simulink model "Control_try_final_2020b"  (R2020b)
settings: Solver=VariableStepAuto  StartTime=0.0  StopTime=inf  RelTol=1e-3
undefined symbols (not defined in the file or in its folder): DiscIntNeverNeededParam
libraries: mobileRoboticsLib x25
(part 3 of 7)

== system Control_try_final_2020b/Team_1_behaviour/T1R3 (defender 1)/Team 1 Behaviour ==
  Ball Loc : Inport
  Robot 1 T1 Loc : Inport  Port=2
  Angle Finder : Subsystem
  Chart : Stateflow chart  TreatAsAtomicUnit=on
      settings: PortSchema="{\"entries\":[{\"content\":{\"sides\":[{\"content\":{\"connectorIds\":[\"In5\",\"In1\",\"In2\",\"In3\",\"In4\",\"In6\"]},\"type\":\"ConnectorPlacement.EquallySpacedRectSide\",\"uuid\":\"cd25ea97-6441-4246-83f2-eec847899c89\"},{\"content\":{\"connectorIds\":[\"Out1\"],\"side\":\"RIGHT\"},\"type\":\"ConnectorPlacement.EquallySpacedRectSide\",\"uuid\":\"ef7d77a7-1549-4474-8b84-35bb8af5d0e7\"},{\"content\":{\"connectorIds\":[],\"side\":\"TOP\"},\"type\":\"ConnectorPlacement.EquallySpacedRectSide\",\"uuid\":\"0f0ce596-3061-42ac-890a-62bc4f21ac3e\"},{\"content\":{\"connectorIds\":[],\"side\":\"BOTTOM\"},\"type\":\"ConnectorPlacement.EquallySpacedRectSide\",\"uuid\":\"682b3de5-e999-4954-b7ff-f16ecbf9ea8f\"}]},\"type\":\"ConnectorPlacement.EquallySpacedConnector\",\"uuid\":\"15dca8e2-6a60-4a0d-80a5-3c295a61c828\"}],\"packageUris\":[\"http://schema.mathworks.com/mf0/Connector/R2020b\"],\"version\":\"1.0\"}"
  Chart3 : Stateflow chart  TreatAsAtomicUnit=on
  Constant : Constant  Value=10
  Constant1 : Constant  Value=4
  Constant2 : Constant  Value=2
  Constant3 : Constant  Value=0
  Demux1 : Demux  Outputs=3
  Demux3 : Demux  Outputs=3
  Matrix Concatenate : Concatenate  Mode=Multidimensional array  ConcatenateDimension=2
  Mod : Math  Operator=mod  SaturateOnIntegerOverflow=on
  Pi : Constant  Value=pi  OutDataTypeStr=Inherit: Inherit via back propagation
  Product1 : Product
  Proximity_Finder_Ball : Subsystem
  Sum : Sum  Inputs=+-
  Sum1 : Sum  Inputs=-+
  Vector Concatenate : Concatenate
  Vector Concatenate1 : Concatenate  NumInputs=3
  Vector Concatenate2 : Concatenate
  Velocity_Decider : Stateflow chart  TreatAsAtomicUnit=on
  kick_direction : Subsystem
  XYZK : Outport
  VxVyW : Outport  Port=2
  wires:
  Ball Loc/1 -> Demux3/1
  Sum/1 -> Proximity_Finder_Ball/1(In1), Angle Finder/1(In1)
  Robot 1 T1 Loc/1 -> Demux1/1
  Demux1/1 -> Matrix Concatenate/1, Chart/3(Rx)
  Demux1/2 -> Matrix Concatenate/2, Chart/4(Ry)
  Matrix Concatenate/1 -> Sum1/2, Sum/1
  Demux3/2 -> Vector Concatenate2/2, Chart/2(By)
  Demux3/1 -> Vector Concatenate2/1, Chart/1(Bx)
  Demux1/3 -> Mod/1
  Pi/1 -> Product1/1
  Constant2/1 -> Product1/2
  Product1/1 -> Mod/2
  Chart/1(actual_angle) -> Chart3/2(DT)
  Mod/1 -> Chart/6(angle_bot)
  Angle Finder/1(angle) -> Chart/5(angle)
  Proximity_Finder_Ball/1(DBR) -> Velocity_Decider/1(DBR)
  Velocity_Decider/2(velocity) -> Chart3/1(velocity)
  Constant/1 -> Vector Concatenate/1
  Constant1/1 -> Vector Concatenate/2
  Vector Concatenate/1 -> Sum1/1
  Sum1/1 -> kick_direction/1(In1)
  Velocity_Decider/1(kick) -> kick_direction/2(kick)
  kick_direction/1(Out1) -> XYZK/1
  Chart3/1(v) -> Vector Concatenate1/1
  Chart3/2(w) -> Vector Concatenate1/3
  Constant3/1 -> Vector Concatenate1/2
  Vector Concatenate1/1 -> VxVyW/1
  Vector Concatenate2/1 -> Sum/2

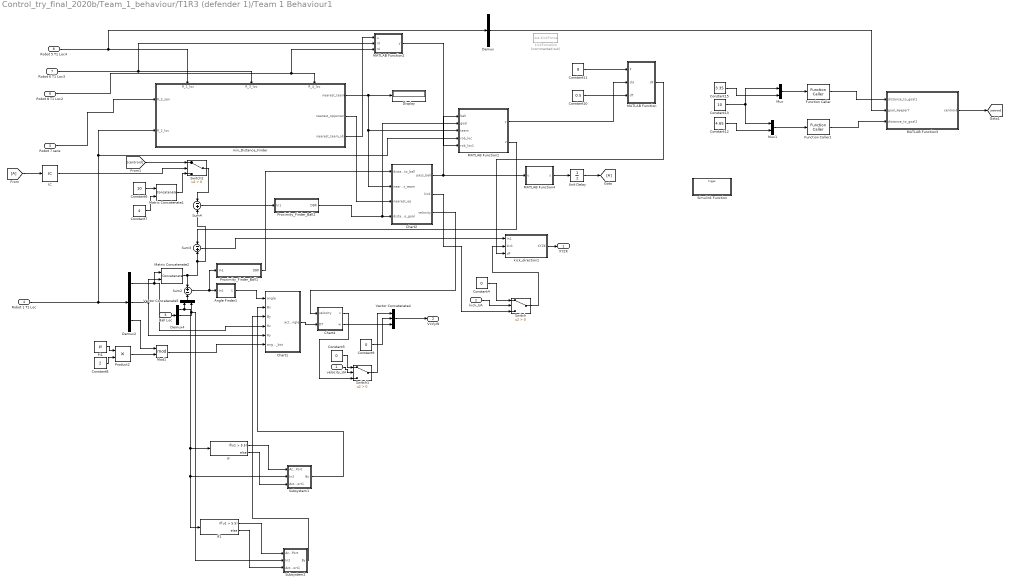
== system Control_try_final_2020b/Team_1_behaviour/T1R3 (defender 1)/Team 1 Behaviour1 ==
  velocity_UA : Inport
  kick_UA : Inport  Port=2
  Ball Loc : Inport  Port=3
  Robot 1 T1 Loc : Inport  Port=4
  Robot 7 sens : Inport  Port=5
  Robot 8 T1 Loc2 : Inport  Port=6
  Robot 6 T1 Loc3 : Inport  Port=7
  Robot 5 T1 Loc4 : Inport  Port=8
  Angle Finder1 : Subsystem
  Chart1 : Stateflow chart  TreatAsAtomicUnit=on
      settings: PortSchema="{\"entries\":[{\"content\":{\"sides\":[{\"content\":{\"connectorIds\":[\"In5\",\"In1\",\"In2\",\"In3\",\"In4\",\"In6\"]},\"type\":\"ConnectorPlacement.EquallySpacedRectSide\",\"uuid\":\"cd25ea97-6441-4246-83f2-eec847899c89\"},{\"content\":{\"connectorIds\":[\"Out1\"],\"side\":\"RIGHT\"},\"type\":\"ConnectorPlacement.EquallySpacedRectSide\",\"uuid\":\"ef7d77a7-1549-4474-8b84-35bb8af5d0e7\"},{\"content\":{\"connectorIds\":[],\"side\":\"TOP\"},\"type\":\"ConnectorPlacement.EquallySpacedRectSide\",\"uuid\":\"0f0ce596-3061-42ac-890a-62bc4f21ac3e\"},{\"content\":{\"connectorIds\":[],\"side\":\"BOTTOM\"},\"type\":\"ConnectorPlacement.EquallySpacedRectSide\",\"uuid\":\"682b3de5-e999-4954-b7ff-f16ecbf9ea8f\"}]},\"type\":\"ConnectorPlacement.EquallySpacedConnector\",\"uuid\":\"15dca8e2-6a60-4a0d-80a5-3c295a61c828\"}],\"packageUris\":[\"http://schema.mathworks.com/mf0/Connector/R2020b\"],\"version\":\"1.0\"}"
  Chart2 : Stateflow chart  TreatAsAtomicUnit=on
      settings: PortSchema="{\"entries\":[{\"content\":{\"sides\":[{\"content\":{\"connectorIds\":[\"In1\",\"In2\",\"In3\",\"In4\"]},\"type\":\"ConnectorPlacement.EquallySpacedRectSide\",\"uuid\":\"0588d813-8053-43c2-aa9d-d3a846613814\"},{\"content\":{\"connectorIds\":[\"Out3\",\"Out1\",\"Out2\"],\"side\":\"RIGHT\"},\"type\":\"ConnectorPlacement.EquallySpacedRectSide\",\"uuid\":\"b273383a-6a54-4b9f-9eb1-40fc7adfc00e\"},{\"content\":{\"connectorIds\":[],\"side\":\"TOP\"},\"type\":\"ConnectorPlacement.EquallySpacedRectSide\",\"uuid\":\"d9b37716-6c8a-415a-a248-7c4c2a5acdca\"}]},\"type\":\"ConnectorPlacement.EquallySpacedConnector\",\"uuid\":\"4383e6fa-6fc5-4afb-a6cc-0c4f83dd9bd6\"}],\"packageUris\":[\"http://schema.mathworks.com/mf0/Connector/R2020b\"],\"version\":\"1.0\"}"
  Chart4 : Stateflow chart  TreatAsAtomicUnit=on
  Constant10 : Constant  Value=0.5
  Constant11 : Constant  Value=8
  Constant12 : Constant  Value=4.65
  Constant13 : Constant  Value=10
  Constant15 : Constant  Value=3.35
  Constant4 : Constant  Value=0
  Constant5 : Constant  Value=0
  Constant6 : Constant  Value=10
  Constant7 : Constant  Value=4
  Constant8 : Constant  Value=2
  Constant9 : Constant  Value=0
  Demux : Demux  Outputs=3
  Demux2 : Demux  Outputs=3
  Demux4 : Demux  Outputs=3
  Display : Display
  Function Caller : FunctionCaller  FunctionPrototype=y = f(u)  InputArgumentSpecifications=<Enter example>  OutputArgumentSpecifications=<Enter example>
  Function Caller1 : FunctionCaller  FunctionPrototype=y = f(u)  InputArgumentSpecifications=<Enter example>  OutputArgumentSpecifications=<Enter example>
  IC : InitialCondition  Value=0
  If : If  IfExpression=u1 > 5.5
  If1 : If  IfExpression=u1 > 5.5
  MATLAB Function : MATLAB Function  TreatAsAtomicUnit=on
  MATLAB Function1 : MATLAB Function  TreatAsAtomicUnit=on
  MATLAB Function2 : MATLAB Function  TreatAsAtomicUnit=on
  MATLAB Function3 : MATLAB Function  TreatAsAtomicUnit=on
  MATLAB Function4 : MATLAB Function  TreatAsAtomicUnit=on
  Matrix Concatenate1 : Concatenate  Mode=Multidimensional array  ConcatenateDimension=2
  Matrix Concatenate2 : Concatenate  Mode=Multidimensional array  ConcatenateDimension=2
  Mod1 : Math  Operator=mod  SaturateOnIntegerOverflow=on
  Mux : Mux  Inputs=2
  Mux1 : Mux  Inputs=2
  Pi1 : Constant  Value=pi  OutDataTypeStr=Inherit: Inherit via back propagation
  Product2 : Product
  Proximity_Finder_Ball1 : Subsystem
  Proximity_Finder_Ball2 : Subsystem
  Simulink Function : Subsystem  TreatAsAtomicUnit=on
  Subsystem1 : Subsystem
  Subsystem2 : Subsystem
  Sum2 : Sum  Inputs=+-
  Sum3 : Sum  Inputs=-+
  Sum4 : Sum  Inputs=-+
  Switch : Switch  Criteria=u2 > Threshold
  Switch1 : Switch  Criteria=u2 > Threshold
  Switch2 : Switch  Criteria=u2 > Threshold
  Unit Delay : UnitDelay  SampleTime=-1  HasFrameUpgradeWarning=on
  Vector Concatenate4 : Concatenate  NumInputs=3
  Vector Concatenate5 : Concatenate
  kickForceSim : FromWorkspace  Commented=on  VariableName=out.KickForce
  kick_direction1 : Subsystem
  min_Distance_Finder : Subsystem
      settings: PortSchema="{\"entries\":[{\"content\":{\"sides\":[{\"content\":{\"connectorIds\":[\"In1\",\"In2\"]},\"type\":\"ConnectorPlacement.EquallySpacedRectSide\",\"uuid\":\"45cf91c7-7d38-4a19-bf35-d1d31095287a\"},{\"content\":{\"connectorIds\":[\"Out1\",\"Out2\",\"Out3\"],\"side\":\"RIGHT\"},\"type\":\"ConnectorPlacement.EquallySpacedRectSide\",\"uuid\":\"645394ba-2e5d-4060-b61c-cc9330ee0038\"},{\"content\":{\"connectorIds\":[\"In3\",\"In4\",\"In5\"],\"side\":\"TOP\"},\"type\":\"ConnectorPlacement.EquallySpacedRectSide\",\"uuid\":\"4fc56b73-04ec-476f-b487-f0e593f708ad\"},{\"content\":{\"connectorIds\":[],\"side\":\"BOTTOM\"},\"type\":\"ConnectorPlacement.EquallySpacedRectSide\",\"uuid\":\"cd306436-fd63-4e79-88e6-7a63c0840ed7\"}]},\"type\":\"ConnectorPlacement.EquallySpacedConnector\",\"uuid\":\"5cf2ee04-00eb-490b-958c-5fb90b43d325\"}],\"packageUris\":[\"http://schema.mathworks.com/mf0/Connector/R2020b\"],\"version\":\"1.0\"}"
  XYZK : Outport
  VxVyW : Outport  Port=2
  wires:
  Constant4/1 -> Switch/1
  kick_UA/1 -> Switch/2
  Constant5/1 -> Switch1/1
  velocity_UA/1 -> Switch1/2
  MATLAB Function4/1(y) -> Unit Delay/1
  If1/2 -> Subsystem2/3(Action Port1)
  Constant6/1 -> Matrix Concatenate1/1
  Constant9/1 -> Vector Concatenate4/2
  Demux4/1 -> If1/1, Subsystem1/2(In2), If/1, Vector Concatenate5/1
  Matrix Concatenate2/1 -> Sum4/2, Sum3/2, Sum2/1
  Chart1/1(actual_angle) -> Chart4/2(DT)
  Subsystem1/1(Bx) -> Chart1/1(Bx)
  Demux2/3 -> Mod1/1
  Constant8/1 -> Product2/2
  If/2 -> Subsystem1/3(Action Port1)
  Sum3/1 -> kick_direction1/1(In1)
  Robot 6 T1 Loc3/1 -> MATLAB Function2/2(r3), min_Distance_Finder/4(R_3_loc)
  Demux4/2 -> Subsystem2/2(In2), Vector Concatenate5/2
  Proximity_Finder_Ball2/1(DBR) -> MATLAB Function1/2(goal), Chart2/4(distance_to_goal)
  min_Distance_Finder/3(nearest_team_idx) -> MATLAB Function2/1(u)
  If1/1 -> Subsystem2/1(Action Port)
  If/1 -> Subsystem1/1(Action Port)
  Pi1/1 -> Product2/1
  Function Caller1/1 -> MATLAB Function3/3(distance_to_goal2)
  Chart4/2(w) -> Vector Concatenate4/3
  Ball Loc/1 -> Demux4/1
  Robot 8 T1 Loc2/1 -> MATLAB Function2/3(r4), min_Distance_Finder/5(R_4_loc)
  [A] -> IC/1
  kick_direction1/1(XYZK) -> XYZK/1
  Robot 7 sens/1 -> min_Distance_Finder/1(R_2_sen)
  Constant15/1 -> Mux/2
  Mod1/1 -> Chart1/6(angle_bot)
  Sum2/1 -> Proximity_Finder_Ball1/1(In1), Angle Finder1/1(In1)
  Robot 1 T1 Loc/1 -> MATLAB Function1/4(rob_loc), min_Distance_Finder/2(R_2_loc), Demux2/1
  Demux/2 -> MATLAB Function3/2(goal_keeperY)
  Constant13/1 -> Mux1/1, Mux/1
  MATLAB Function1/1(y) -> MATLAB Function/2(dis)
  Demux2/2 -> Matrix Concatenate2/2, Chart1/4(Ry)
  MATLAB Function1/2(z) -> Sum3/1
  Unit Delay/1 -> [A]
  Chart2/3(pass_beh) -> MATLAB Function1/1(beh), MATLAB Function4/1(u)
  Vector Concatenate4/1 -> VxVyW/1
  Constant12/1 -> Mux1/2
  Proximity_Finder_Ball1/1(DBR) -> Chart2/1(distance_to_ball)
  Mux1/1 -> Function Caller1/1
  Mux/1 -> Function Caller/1
  Constant10/1 -> MATLAB Function/3(dT)
  Sum4/1 -> Proximity_Finder_Ball2/1(In1)
  MATLAB Function3/1(centroid) -> [centroid]
  Switch2/1 -> Sum4/1
  min_Distance_Finder/1(nearest_team) -> Chart2/2(nearest_team), MATLAB Function1/3(team), Display/1
  min_Distance_Finder/2(nearest_opponent) -> Chart2/3(nearest_op)
  Chart4/1(v) -> Switch1/3
  Chart2/2(velocity) -> Chart4/1(velocity)
  Subsystem2/1(By) -> Chart1/2(By)
  Chart2/1(kick) -> Switch/3
  Function Caller/1 -> MATLAB Function3/1(distance_to_goal1)
  Angle Finder1/1(angle) -> Chart1/5(angle)
  Product2/1 -> Mod1/2
  MATLAB Function/1(dF) -> kick_direction1/3(dF)
  Matrix Concatenate1/1 -> Switch2/3
  Robot 5 T1 Loc4/1 -> Demux/1, min_Distance_Finder/3(R_1_loc)
  MATLAB Function2/1(y) -> MATLAB Function1/5(rob_loc1)
  Constant11/1 -> MATLAB Function/1(F)
  Demux2/1 -> Matrix Concatenate2/1, Chart1/3(Rx)
  Constant7/1 -> Matrix Concatenate1/2
  IC/1 -> Switch2/2
  Vector Concatenate5/1 -> Sum2/2
  [centroid] -> Switch2/1
  Switch/1 -> kick_direction1/2(kick)
  Switch1/1 -> Vector Concatenate4/1

== system Control_try_final_2020b/Team_2_Behaviour/T2_R1(Goal_Keeper)/Distance ==
  In1 : Inport
  In2 : Inport  Port=2
  In3 : Inport  Port=3
  In4 : Inport  Port=4
  Square : Math  Operator=square  SaturateOnIntegerOverflow=on
  Square Root : Sqrt  SaturateOnIntegerOverflow=on
  Square1 : Math  Operator=square  SaturateOnIntegerOverflow=on
  Sum : Sum  Inputs=|+-
  Sum1 : Sum  Inputs=|+-
  Sum2 : Sum  Inputs=|++
  GB_dist : Outport
  wires:
  Square1/1 -> Sum2/2
  Sum2/1 -> Square Root/1
  Square/1 -> Sum2/1
  Sum1/1 -> Square1/1
  Sum/1 -> Square/1
  In1/1 -> Sum/1
  In3/1 -> Sum/2
  In2/1 -> Sum1/1
  In4/1 -> Sum1/2
  Square Root/1 -> GB_dist/1

== system Control_try_final_2020b/Team_2_Behaviour/T2_R1(Goal_Keeper)/angle_finder ==
  kick_direction : Inport
  R_1_loc : Inport  Port=2
  kick : Inport  Port=3
  Atan : Trigonometry  Operator=atan
  Constant : Constant  Value=2.5
  Constant1 : Constant  Value=-2.5
  Constant2 : Constant  Value=0
  Constant3 : Constant  Value=-1
  Cos : Trigonometry  Operator=cos
  Demux : Demux  Outputs=3
  Divide : Product  Inputs=/*
  Product : Product  Inputs=3
  Product1 : Product
  Sin : Trigonometry
  Sum : Sum  Inputs=|+-
  Vector Concatenate : Concatenate  NumInputs=4
  Out1 : Outport
  wires:
  kick_direction/1 -> Sum/1
  R_1_loc/1 -> Sum/2
  Sum/1 -> Demux/1
  Demux/1 -> Divide/1
  Demux/2 -> Divide/2
  Divide/1 -> Atan/1
  Atan/1 -> Cos/1, Sin/1
  Constant/1 -> Product/2
  Cos/1 -> Product/3
  Sin/1 -> Product1/1
  Constant1/1 -> Product1/2
  Vector Concatenate/1 -> Out1/1
  kick/1 -> Vector Concatenate/4
  Constant2/1 -> Vector Concatenate/3
  Product1/1 -> Vector Concatenate/2
  Product/1 -> Vector Concatenate/1
  Constant3/1 -> Product/1

== system Control_try_final_2020b/Team_2_Behaviour/T2_R1(Goal_Keeper)/min_Distance_Finder ==
  R_1_sen : Inport
  R_1_loc : Inport  Port=2
  R_2_loc : Inport  Port=3
  R_3_loc : Inport  Port=4
  R_4_loc : Inport  Port=5
  Display{,1..2,4} (4 alike) : Display
  Distance : Subsystem
  Distance1 : Subsystem
  Distance2 : Subsystem
  Kick_prob_calc : Stateflow chart  TreatAsAtomicUnit=on
      settings: PortSchema="{\"entries\":[{\"content\":{\"sides\":[{\"content\":{\"connectorIds\":[\"In4\",\"In5\",\"In6\"]},\"type\":\"ConnectorPlacement.EquallySpacedRectSide\",\"uuid\":\"64545375-395a-4478-8a53-b77c7ccd5016\"},{\"content\":{\"connectorIds\":[\"Out1\"],\"side\":\"RIGHT\"},\"type\":\"ConnectorPlacement.EquallySpacedRectSide\",\"uuid\":\"7cc0c28a-cc26-4f23-9952-6261e736221a\"},{\"content\":{\"connectorIds\":[\"In2\",\"In3\",\"In1\"],\"side\":\"TOP\"},\"type\":\"ConnectorPlacement.EquallySpacedRectSide\",\"uuid\":\"3f39c863-1804-4707-87c1-6f77798d874b\"},{\"content\":{\"connectorIds\":[],\"side\":\"BOTTOM\"},\"type\":\"ConnectorPlacement.EquallySpacedRectSide\",\"uuid\":\"dd00a5df-2ac1-49a5-bc9d-cbc3bc53305b\"}]},\"type\":\"ConnectorPlacement.EquallySpacedConnector\",\"uuid\":\"731ad359-9b43-4c19-839e-d6f1a372c8a6\"}],\"packageUris\":[\"http://schema.mathworks.com/mf0/Connector/R2020b\"],\"version\":\"1.0\"}"
  Multiply : Gain  Gain=2
  Multiply1 : Gain  Gain=2
  Multiply2 : Gain  Gain=2
  R2_O_dist_val : Subsystem
  R3_O_dist_val : Subsystem
  R4_O_dist_val : Subsystem
  Sum : Sum  Inputs=|--
  Sum1 : Sum  Inputs=|--
  Sum2 : Sum  Inputs=|--
  zero_padding : MATLAB Function  TreatAsAtomicUnit=on
  kick_direction : Outport
  wires:
  R_2_loc/1 -> R2_O_dist_val/2(R_2_loc), Distance/2(R_2_loc), Kick_prob_calc/2(R_2_loc)
  R_1_loc/1 -> R4_O_dist_val/1(R_1_loc), R3_O_dist_val/1(R_1_loc), R2_O_dist_val/1(R_1_loc), Distance2/1(R_1_loc), Distance1/1(R_1_loc), Distance/1(R_1_loc)
  R_3_loc/1 -> R3_O_dist_val/2(R_2_loc), Distance1/2(R_3_loc), Kick_prob_calc/3(R_3_loc)
  R_4_loc/1 -> R4_O_dist_val/2(R_2_loc), Distance2/2(R_4_loc), Kick_prob_calc/1(R_4_loc)
  Kick_prob_calc/1(kick_direction) -> Display4/1, kick_direction/1
  R_1_sen/1 -> zero_padding/1(u)
  zero_padding/1(y) -> R3_O_dist_val/3(sen_1_val), R4_O_dist_val/3(sen_1_val), R2_O_dist_val/3(sen_1_val)
  R2_O_dist_val/1(y) -> Display/1, Multiply1/1
  R3_O_dist_val/1(y) -> Display1/1, Multiply2/1
  R4_O_dist_val/1(y) -> Display2/1, Multiply/1
  Distance/1(R1_R2_dis) -> Sum/1
  Multiply1/1 -> Sum/2
  Distance1/1(R1_R3_dis) -> Sum1/1
  Distance2/1(R1_R4_dis) -> Sum2/1
  Multiply2/1 -> Sum1/2
  Multiply/1 -> Sum2/2
  Sum/1 -> Kick_prob_calc/4(R1_R2_dis)
  Sum1/1 -> Kick_prob_calc/5(R1_R3_dis)
  Sum2/1 -> Kick_prob_calc/6(R1_R4_dis)

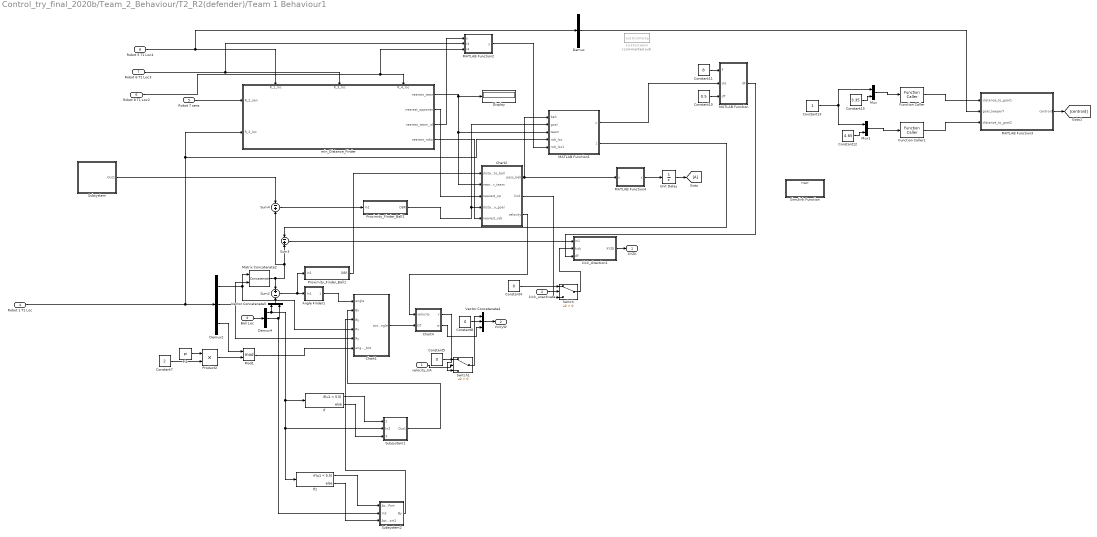
== system Control_try_final_2020b/Team_2_Behaviour/T2_R2(defender)/Team 1 Behaviour1 ==
  velocity_UA : Inport
  kick_unactivate : Inport  Port=2
  Ball Loc : Inport  Port=3
  Robot 1 T1 Loc : Inport  Port=4
  Robot 7 sens : Inport  Port=5
  Robot 8 T1 Loc2 : Inport  Port=6
  Robot 6 T1 Loc3 : Inport  Port=7
  Robot 5 T1 Loc4 : Inport  Port=8
  Angle Finder1 : Subsystem
  Chart1 : Stateflow chart  TreatAsAtomicUnit=on
      settings: PortSchema="{\"entries\":[{\"content\":{\"sides\":[{\"content\":{\"connectorIds\":[\"In5\",\"In1\",\"In2\",\"In3\",\"In4\",\"In6\"]},\"type\":\"ConnectorPlacement.EquallySpacedRectSide\",\"uuid\":\"cd25ea97-6441-4246-83f2-eec847899c89\"},{\"content\":{\"connectorIds\":[\"Out1\"],\"side\":\"RIGHT\"},\"type\":\"ConnectorPlacement.EquallySpacedRectSide\",\"uuid\":\"ef7d77a7-1549-4474-8b84-35bb8af5d0e7\"},{\"content\":{\"connectorIds\":[],\"side\":\"TOP\"},\"type\":\"ConnectorPlacement.EquallySpacedRectSide\",\"uuid\":\"0f0ce596-3061-42ac-890a-62bc4f21ac3e\"},{\"content\":{\"connectorIds\":[],\"side\":\"BOTTOM\"},\"type\":\"ConnectorPlacement.EquallySpacedRectSide\",\"uuid\":\"682b3de5-e999-4954-b7ff-f16ecbf9ea8f\"}]},\"type\":\"ConnectorPlacement.EquallySpacedConnector\",\"uuid\":\"15dca8e2-6a60-4a0d-80a5-3c295a61c828\"}],\"packageUris\":[\"http://schema.mathworks.com/mf0/Connector/R2020b\"],\"version\":\"1.0\"}"
  Chart2 : Stateflow chart  TreatAsAtomicUnit=on
      settings: PortSchema="{\"entries\":[{\"content\":{\"sides\":[{\"content\":{\"connectorIds\":[\"In1\",\"In2\",\"In3\",\"In4\",\"In5\"]},\"type\":\"ConnectorPlacement.EquallySpacedRectSide\",\"uuid\":\"0588d813-8053-43c2-aa9d-d3a846613814\"},{\"content\":{\"connectorIds\":[\"Out3\",\"Out1\",\"Out2\"],\"side\":\"RIGHT\"},\"type\":\"ConnectorPlacement.EquallySpacedRectSide\",\"uuid\":\"b273383a-6a54-4b9f-9eb1-40fc7adfc00e\"},{\"content\":{\"connectorIds\":[],\"side\":\"TOP\"},\"type\":\"ConnectorPlacement.EquallySpacedRectSide\",\"uuid\":\"d9b37716-6c8a-415a-a248-7c4c2a5acdca\"}]},\"type\":\"ConnectorPlacement.EquallySpacedConnector\",\"uuid\":\"4383e6fa-6fc5-4afb-a6cc-0c4f83dd9bd6\"}],\"packageUris\":[\"http://schema.mathworks.com/mf0/Connector/R2020b\"],\"version\":\"1.0\"}"
  Chart4 : Stateflow chart  TreatAsAtomicUnit=on
  Constant10 : Constant  Value=0.5
  Constant11 : Constant  Value=8
  Constant12 : Constant  Value=4.65
  Constant13 : Constant
  Constant15 : Constant  Value=3.35
  Constant4 : Constant  Value=0
  Constant5 : Constant  Value=0
  Constant7 : Constant  Value=2
  Constant8 : Constant  Value=0
  Demux : Demux  Outputs=3
  Demux2 : Demux  Outputs=3
  Demux4 : Demux  Outputs=3
  Display : Display
  Function Caller : FunctionCaller  FunctionPrototype=y = f(u)  InputArgumentSpecifications=<Enter example>  OutputArgumentSpecifications=<Enter example>
  Function Caller1 : FunctionCaller  FunctionPrototype=y = f(u)  InputArgumentSpecifications=<Enter example>  OutputArgumentSpecifications=<Enter example>
  If : If  IfExpression=u1 < 5.5
  If1 : If  IfExpression=u1 < 5.5
  MATLAB Function : MATLAB Function  TreatAsAtomicUnit=on
  MATLAB Function1 : MATLAB Function  TreatAsAtomicUnit=on
  MATLAB Function2 : MATLAB Function  TreatAsAtomicUnit=on
  MATLAB Function3 : MATLAB Function  TreatAsAtomicUnit=on
  MATLAB Function4 : MATLAB Function  TreatAsAtomicUnit=on
  Matrix Concatenate2 : Concatenate  Mode=Multidimensional array  ConcatenateDimension=2
  Mod1 : Math  Operator=mod  SaturateOnIntegerOverflow=on
  Mux : Mux  Inputs=2
  Mux1 : Mux  Inputs=2
  Pi1 : Constant  Value=pi  OutDataTypeStr=Inherit: Inherit via back propagation
  Product2 : Product
  Proximity_Finder_Ball1 : Subsystem
  Proximity_Finder_Ball2 : Subsystem
  Simulink Function : Subsystem  TreatAsAtomicUnit=on
  Subsystem : Subsystem
  Subsystem1 : Subsystem
  Subsystem2 : Subsystem
  Sum2 : Sum  Inputs=+-
  Sum3 : Sum  Inputs=-+
  Sum4 : Sum  Inputs=-+
  Switch : Switch  Criteria=u2 > Threshold
  Switch1 : Switch  Criteria=u2 > Threshold
  Unit Delay : UnitDelay  SampleTime=-1  HasFrameUpgradeWarning=on
  Vector Concatenate4 : Concatenate  NumInputs=3
  Vector Concatenate5 : Concatenate
  kickForceSim : FromWorkspace  Commented=on  VariableName=out.KickForce
  kick_direction1 : Subsystem
  min_Distance_Finder : Subsystem
      settings: PortSchema="{\"entries\":[{\"content\":{\"sides\":[{\"content\":{\"connectorIds\":[\"In1\",\"In2\"]},\"type\":\"ConnectorPlacement.EquallySpacedRectSide\",\"uuid\":\"45cf91c7-7d38-4a19-bf35-d1d31095287a\"},{\"content\":{\"connectorIds\":[\"Out1\",\"Out2\",\"Out3\",\"Out4\"],\"side\":\"RIGHT\"},\"type\":\"ConnectorPlacement.EquallySpacedRectSide\",\"uuid\":\"645394ba-2e5d-4060-b61c-cc9330ee0038\"},{\"content\":{\"connectorIds\":[\"In3\",\"In4\",\"In5\"],\"side\":\"TOP\"},\"type\":\"ConnectorPlacement.EquallySpacedRectSide\",\"uuid\":\"4fc56b73-04ec-476f-b487-f0e593f708ad\"},{\"content\":{\"connectorIds\":[],\"side\":\"BOTTOM\"},\"type\":\"ConnectorPlacement.EquallySpacedRectSide\",\"uuid\":\"cd306436-fd63-4e79-88e6-7a63c0840ed7\"}]},\"type\":\"ConnectorPlacement.EquallySpacedConnector\",\"uuid\":\"5cf2ee04-00eb-490b-958c-5fb90b43d325\"}],\"packageUris\":[\"http://schema.mathworks.com/mf0/Connector/R2020b\"],\"version\":\"1.0\"}"
  XYZK : Outport
  VxVyW : Outport  Port=2
  wires:
  Constant4/1 -> Switch/1
  kick_unactivate/1 -> Switch/2
  Constant5/1 -> Switch1/1
  velocity_UA/1 -> Switch1/2
  Constant7/1 -> Product2/2
  Subsystem1/1(Out1) -> Chart1/1(Bx)
  min_Distance_Finder/3(nearest_team_idx) -> MATLAB Function2/1(u)
  Sum4/1 -> Proximity_Finder_Ball2/1(In1)
  If1/2 -> Subsystem2/3(Action Port1)
  MATLAB Function1/2(z) -> Sum3/1
  Robot 7 sens/1 -> min_Distance_Finder/1(R_2_sen)
  Mod1/1 -> Chart1/6(angle_bot)
  Sum2/1 -> Proximity_Finder_Ball1/1(In1), Angle Finder1/1(In1)
  Function Caller/1 -> MATLAB Function3/1(distance_to_goal1)
  Robot 8 T1 Loc2/1 -> MATLAB Function2/3(r4), min_Distance_Finder/5(R_4_loc)
  MATLAB Function/1(dF) -> kick_direction1/3(dF)
  Robot 1 T1 Loc/1 -> MATLAB Function1/4(rob_loc), min_Distance_Finder/2(R_2_loc), Demux2/1
  If/2 -> Subsystem1/3(Action Port1)
  Constant12/1 -> Mux1/2
  Demux4/2 -> Subsystem2/2(In2), Vector Concatenate5/2
  Vector Concatenate5/1 -> Sum2/2
  MATLAB Function3/1(centroid) -> [centroid]
  MATLAB Function1/1(y) -> MATLAB Function/2(dis)
  MATLAB Function4/1(y) -> Unit Delay/1
  Constant11/1 -> MATLAB Function/1(F)
  Robot 6 T1 Loc3/1 -> MATLAB Function2/2(r3), min_Distance_Finder/4(R_3_loc)
  Constant8/1 -> Vector Concatenate4/2
  Constant10/1 -> MATLAB Function/3(dT)
  Proximity_Finder_Ball2/1(DBR) -> MATLAB Function1/2(goal), Chart2/4(distance_to_goal)
  Sum3/1 -> kick_direction1/1(In1)
  Demux/2 -> MATLAB Function3/2(goal_keeperY)
  Chart4/1(v) -> Switch1/3
  Proximity_Finder_Ball1/1(DBR) -> Chart2/1(distance_to_ball)
  min_Distance_Finder/4(nearest_robot) -> Chart2/5(nearest_rob)
  Unit Delay/1 -> [A]
  Subsystem2/1(By) -> Chart1/2(By)
  kick_direction1/1(XYZK) -> XYZK/1
  Demux4/1 -> Vector Concatenate5/1, If1/1, Subsystem1/2(In2), If/1
  Mux/1 -> Function Caller/1
  Vector Concatenate4/1 -> VxVyW/1
  Constant15/1 -> Mux/2
  MATLAB Function2/1(y) -> MATLAB Function1/5(rob_loc1)
  Robot 5 T1 Loc4/1 -> Demux/1, min_Distance_Finder/3(R_1_loc)
  Pi1/1 -> Product2/1
  Constant13/1 -> Mux1/1, Mux/1
  Matrix Concatenate2/1 -> Sum4/2, Sum3/2, Sum2/1
  Demux2/3 -> Mod1/1
  Subsystem/1(Out1) -> Sum4/1
  If/1 -> Subsystem1/1(Action Port)
  min_Distance_Finder/2(nearest_opponent) -> Chart2/3(nearest_op)
  Chart4/2(w) -> Vector Concatenate4/3
  Chart2/3(pass_beh) -> MATLAB Function4/1(u), MATLAB Function1/1(beh)
  Product2/1 -> Mod1/2
  Angle Finder1/1(angle) -> Chart1/5(angle)
  Mux1/1 -> Function Caller1/1
  Chart2/2(velocity) -> Chart4/1(velocity)
  Chart1/1(actual_angle) -> Chart4/2(DT)
  Demux2/1 -> Matrix Concatenate2/1, Chart1/3(Rx)
  min_Distance_Finder/1(nearest_team) -> Chart2/2(nearest_team), MATLAB Function1/3(team), Display/1
  Function Caller1/1 -> MATLAB Function3/3(distance_to_goal2)
  Demux2/2 -> Matrix Concatenate2/2, Chart1/4(Ry)
  If1/1 -> Subsystem2/1(Action Port)
  Ball Loc/1 -> Demux4/1
  Chart2/1(kick) -> Switch/3
  Switch/1 -> kick_direction1/2(kick)
  Switch1/1 -> Vector Concatenate4/1

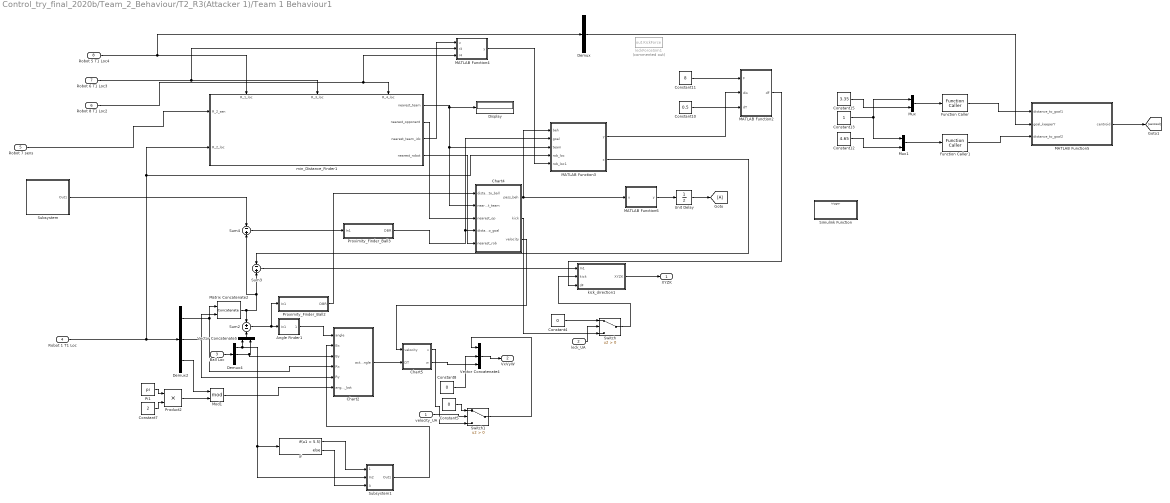
== system Control_try_final_2020b/Team_2_Behaviour/T2_R3(Attacker 1)/Team 1 Behaviour1 ==
  velocity_UA : Inport
  kick_UA : Inport  Port=2
  Ball Loc : Inport  Port=3
  Robot 1 T1 Loc : Inport  Port=4
  Robot 7 sens : Inport  Port=5
  Robot 8 T1 Loc2 : Inport  Port=6
  Robot 6 T1 Loc3 : Inport  Port=7
  Robot 5 T1 Loc4 : Inport  Port=8
  Angle Finder1 : Subsystem
  Chart2 : Stateflow chart  TreatAsAtomicUnit=on
      settings: PortSchema="{\"entries\":[{\"content\":{\"sides\":[{\"content\":{\"connectorIds\":[\"In5\",\"In1\",\"In2\",\"In3\",\"In4\",\"In6\"]},\"type\":\"ConnectorPlacement.EquallySpacedRectSide\",\"uuid\":\"cd25ea97-6441-4246-83f2-eec847899c89\"},{\"content\":{\"connectorIds\":[\"Out1\"],\"side\":\"RIGHT\"},\"type\":\"ConnectorPlacement.EquallySpacedRectSide\",\"uuid\":\"ef7d77a7-1549-4474-8b84-35bb8af5d0e7\"},{\"content\":{\"connectorIds\":[],\"side\":\"TOP\"},\"type\":\"ConnectorPlacement.EquallySpacedRectSide\",\"uuid\":\"0f0ce596-3061-42ac-890a-62bc4f21ac3e\"},{\"content\":{\"connectorIds\":[],\"side\":\"BOTTOM\"},\"type\":\"ConnectorPlacement.EquallySpacedRectSide\",\"uuid\":\"682b3de5-e999-4954-b7ff-f16ecbf9ea8f\"}]},\"type\":\"ConnectorPlacement.EquallySpacedConnector\",\"uuid\":\"15dca8e2-6a60-4a0d-80a5-3c295a61c828\"}],\"packageUris\":[\"http://schema.mathworks.com/mf0/Connector/R2020b\"],\"version\":\"1.0\"}"
  Chart4 : Stateflow chart  TreatAsAtomicUnit=on
      settings: PortSchema="{\"entries\":[{\"content\":{\"sides\":[{\"content\":{\"connectorIds\":[\"In1\",\"In2\",\"In3\",\"In4\",\"In5\"]},\"type\":\"ConnectorPlacement.EquallySpacedRectSide\",\"uuid\":\"0588d813-8053-43c2-aa9d-d3a846613814\"},{\"content\":{\"connectorIds\":[\"Out3\",\"Out1\",\"Out2\"],\"side\":\"RIGHT\"},\"type\":\"ConnectorPlacement.EquallySpacedRectSide\",\"uuid\":\"b273383a-6a54-4b9f-9eb1-40fc7adfc00e\"},{\"content\":{\"connectorIds\":[],\"side\":\"TOP\"},\"type\":\"ConnectorPlacement.EquallySpacedRectSide\",\"uuid\":\"d9b37716-6c8a-415a-a248-7c4c2a5acdca\"}]},\"type\":\"ConnectorPlacement.EquallySpacedConnector\",\"uuid\":\"4383e6fa-6fc5-4afb-a6cc-0c4f83dd9bd6\"}],\"packageUris\":[\"http://schema.mathworks.com/mf0/Connector/R2020b\"],\"version\":\"1.0\"}"
  Chart5 : Stateflow chart  TreatAsAtomicUnit=on
  Constant10 : Constant  Value=0.5
  Constant11 : Constant  Value=8
  Constant12 : Constant  Value=4.65
  Constant13 : Constant
  Constant15 : Constant  Value=3.35
  Constant4 : Constant  Value=0
  Constant5 : Constant  Value=0
  Constant7 : Constant  Value=2
  Constant8 : Constant  Value=0
  Demux : Demux  Outputs=3
  Demux2 : Demux  Outputs=3
  Demux4 : Demux  Outputs=3
  Display : Display
  Function Caller : FunctionCaller  FunctionPrototype=y = f(u)  InputArgumentSpecifications=<Enter example>  OutputArgumentSpecifications=<Enter example>
  Function Caller1 : FunctionCaller  FunctionPrototype=y = f(u)  InputArgumentSpecifications=<Enter example>  OutputArgumentSpecifications=<Enter example>
  If : If  IfExpression=u1 > 5.5
  MATLAB Function2 : MATLAB Function  TreatAsAtomicUnit=on
  MATLAB Function3 : MATLAB Function  TreatAsAtomicUnit=on
  MATLAB Function4 : MATLAB Function  TreatAsAtomicUnit=on
  MATLAB Function5 : MATLAB Function  TreatAsAtomicUnit=on
  MATLAB Function6 : MATLAB Function  TreatAsAtomicUnit=on
  Matrix Concatenate2 : Concatenate  Mode=Multidimensional array  ConcatenateDimension=2
  Mod1 : Math  Operator=mod  SaturateOnIntegerOverflow=on
  Mux : Mux  Inputs=2
  Mux1 : Mux  Inputs=2
  Pi1 : Constant  Value=pi  OutDataTypeStr=Inherit: Inherit via back propagation
  Product2 : Product
  Proximity_Finder_Ball2 : Subsystem
  Proximity_Finder_Ball3 : Subsystem
  Simulink Function : Subsystem  TreatAsAtomicUnit=on
  Subsystem : Subsystem
  Subsystem1 : Subsystem
  Sum2 : Sum  Inputs=+-
  Sum3 : Sum  Inputs=-+
  Sum4 : Sum  Inputs=-+
  Switch : Switch  Criteria=u2 > Threshold
  Switch1 : Switch  Criteria=u2 > Threshold
  Unit Delay : UnitDelay  SampleTime=-1  HasFrameUpgradeWarning=on
  Vector Concatenate4 : Concatenate  NumInputs=3
  Vector Concatenate5 : Concatenate
  kickForceSim1 : FromWorkspace  Commented=on  VariableName=out.KickForce
  kick_direction1 : Subsystem
  min_Distance_Finder1 : Subsystem
      settings: PortSchema="{\"entries\":[{\"content\":{\"sides\":[{\"content\":{\"connectorIds\":[\"In1\",\"In2\"]},\"type\":\"ConnectorPlacement.EquallySpacedRectSide\",\"uuid\":\"45cf91c7-7d38-4a19-bf35-d1d31095287a\"},{\"content\":{\"connectorIds\":[\"Out1\",\"Out2\",\"Out3\",\"Out4\"],\"side\":\"RIGHT\"},\"type\":\"ConnectorPlacement.EquallySpacedRectSide\",\"uuid\":\"645394ba-2e5d-4060-b61c-cc9330ee0038\"},{\"content\":{\"connectorIds\":[\"In3\",\"In4\",\"In5\"],\"side\":\"TOP\"},\"type\":\"ConnectorPlacement.EquallySpacedRectSide\",\"uuid\":\"4fc56b73-04ec-476f-b487-f0e593f708ad\"},{\"content\":{\"connectorIds\":[],\"side\":\"BOTTOM\"},\"type\":\"ConnectorPlacement.EquallySpacedRectSide\",\"uuid\":\"cd306436-fd63-4e79-88e6-7a63c0840ed7\"}]},\"type\":\"ConnectorPlacement.EquallySpacedConnector\",\"uuid\":\"5cf2ee04-00eb-490b-958c-5fb90b43d325\"}],\"packageUris\":[\"http://schema.mathworks.com/mf0/Connector/R2020b\"],\"version\":\"1.0\"}"
  XYZK : Outport
  VxVyW : Outport  Port=2
  wires:
  Constant4/1 -> Switch/1
  kick_UA/1 -> Switch/2
  Constant5/1 -> Switch1/1
  velocity_UA/1 -> Switch1/2
  Sum3/1 -> kick_direction1/1(In1)
  Function Caller1/1 -> MATLAB Function5/3(distance_to_goal2)
  Robot 7 sens/1 -> min_Distance_Finder1/1(R_2_sen)
  Demux4/1 -> Vector Concatenate5/1, Subsystem1/2(In2), If/1
  MATLAB Function4/1(y) -> MATLAB Function3/5(rob_loc1)
  min_Distance_Finder1/4(nearest_robot) -> Chart4/5(nearest_rob)
  Vector Concatenate5/1 -> Sum2/2
  min_Distance_Finder1/3(nearest_team_idx) -> MATLAB Function4/1(u)
  MATLAB Function2/1(dF) -> kick_direction1/3(dF)
  Robot 6 T1 Loc3/1 -> MATLAB Function4/2(r3), min_Distance_Finder1/4(R_3_loc)
  Robot 5 T1 Loc4/1 -> Demux/1, min_Distance_Finder1/3(R_1_loc)
  MATLAB Function5/1(centroid) -> [centroid]
  Sum2/1 -> Proximity_Finder_Ball2/1(In1), Angle Finder1/1(In1)
  Vector Concatenate4/1 -> VxVyW/1
  Subsystem/1(Out1) -> Sum4/1
  Mod1/1 -> Chart2/6(angle_bot)
  Matrix Concatenate2/1 -> Sum4/2, Sum3/2, Sum2/1
  Chart2/1(actual_angle) -> Chart5/2(DT)
  Proximity_Finder_Ball3/1(DBR) -> MATLAB Function3/2(goal), Chart4/4(distance_to_goal)
  Ball Loc/1 -> Demux4/1
  Constant11/1 -> MATLAB Function2/1(F)
  Constant15/1 -> Mux/2
  MATLAB Function3/2(z) -> Sum3/1
  Constant12/1 -> Mux1/2
  Demux/2 -> MATLAB Function5/2(goal_keeperY)
  Unit Delay/1 -> [A]
  Mux/1 -> Function Caller/1
  Constant8/1 -> Vector Concatenate4/2
  Chart4/2(velocity) -> Chart5/1(velocity)
  Robot 1 T1 Loc/1 -> MATLAB Function3/4(rob_loc), min_Distance_Finder1/2(R_2_loc), Demux2/1
  Demux4/2 -> Chart2/2(By), Vector Concatenate5/2
  MATLAB Function3/1(y) -> MATLAB Function2/2(dis)
  Proximity_Finder_Ball2/1(DBR) -> Chart4/1(distance_to_ball)
  Subsystem1/1(Out1) -> Chart2/1(Bx)
  Constant13/1 -> Mux1/1, Mux/1
  kick_direction1/1(XYZK) -> XYZK/1
  If/2 -> Subsystem1/3(Action Port1)
  Constant7/1 -> Product2/2
  Demux2/3 -> Mod1/1
  Demux2/2 -> Matrix Concatenate2/2, Chart2/4(Ry)
  Product2/1 -> Mod1/2
  Constant10/1 -> MATLAB Function2/3(dT)
  Mux1/1 -> Function Caller1/1
  Chart5/2(w) -> Vector Concatenate4/3
  Chart4/3(pass_beh) -> MATLAB Function6/1(u), MATLAB Function3/1(beh)
  MATLAB Function6/1(y) -> Unit Delay/1
  Pi1/1 -> Product2/1
  Function Caller/1 -> MATLAB Function5/1(distance_to_goal1)
  min_Distance_Finder1/2(nearest_opponent) -> Chart4/3(nearest_op)
  Sum4/1 -> Proximity_Finder_Ball3/1(In1)
  Demux2/1 -> Matrix Concatenate2/1, Chart2/3(Rx)
  Angle Finder1/1(angle) -> Chart2/5(angle)
  Robot 8 T1 Loc2/1 -> MATLAB Function4/3(r4), min_Distance_Finder1/5(R_4_loc)
  min_Distance_Finder1/1(nearest_team) -> Chart4/2(nearest_team), MATLAB Function3/3(team), Display/1
  If/1 -> Subsystem1/1(Action Port)
  Chart4/1(kick) -> Switch/3
  Switch/1 -> kick_direction1/2(kick)
  Switch1/1 -> Vector Concatenate4/1
  Chart5/1(v) -> Switch1/3

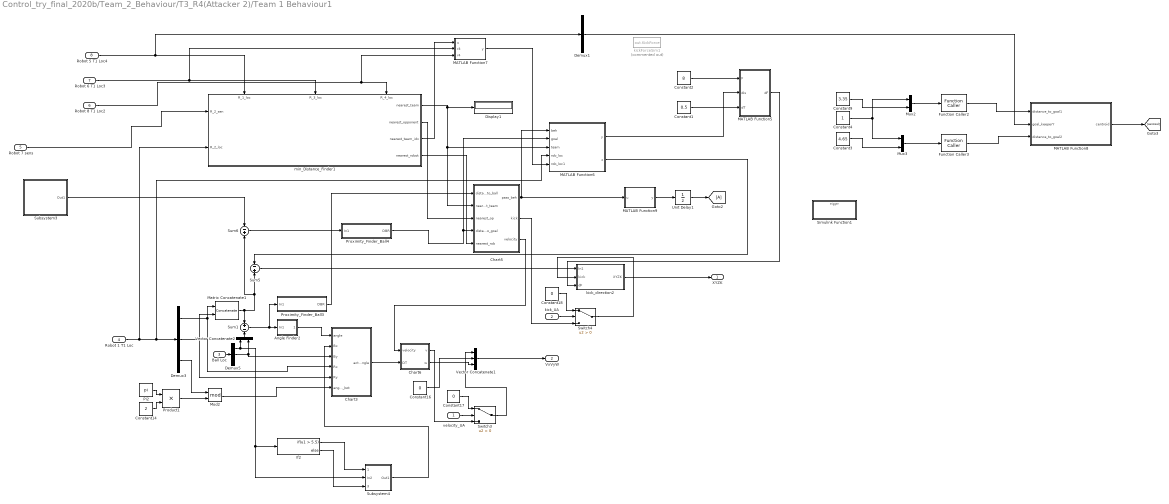
== system Control_try_final_2020b/Team_2_Behaviour/T3_R4(Attacker 2)/Team 1 Behaviour1 ==
  velocity_UA : Inport
  kick_UA : Inport  Port=2
  Ball Loc : Inport  Port=3
  Robot 1 T1 Loc : Inport  Port=4
  Robot 7 sens : Inport  Port=5
  Robot 8 T1 Loc2 : Inport  Port=6
  Robot 6 T1 Loc3 : Inport  Port=7
  Robot 5 T1 Loc4 : Inport  Port=8
  Angle Finder2 : Subsystem
  Chart3 : Stateflow chart  TreatAsAtomicUnit=on
      settings: PortSchema="{\"entries\":[{\"content\":{\"sides\":[{\"content\":{\"connectorIds\":[\"In5\",\"In1\",\"In2\",\"In3\",\"In4\",\"In6\"]},\"type\":\"ConnectorPlacement.EquallySpacedRectSide\",\"uuid\":\"cd25ea97-6441-4246-83f2-eec847899c89\"},{\"content\":{\"connectorIds\":[\"Out1\"],\"side\":\"RIGHT\"},\"type\":\"ConnectorPlacement.EquallySpacedRectSide\",\"uuid\":\"ef7d77a7-1549-4474-8b84-35bb8af5d0e7\"},{\"content\":{\"connectorIds\":[],\"side\":\"TOP\"},\"type\":\"ConnectorPlacement.EquallySpacedRectSide\",\"uuid\":\"0f0ce596-3061-42ac-890a-62bc4f21ac3e\"},{\"content\":{\"connectorIds\":[],\"side\":\"BOTTOM\"},\"type\":\"ConnectorPlacement.EquallySpacedRectSide\",\"uuid\":\"682b3de5-e999-4954-b7ff-f16ecbf9ea8f\"}]},\"type\":\"ConnectorPlacement.EquallySpacedConnector\",\"uuid\":\"15dca8e2-6a60-4a0d-80a5-3c295a61c828\"}],\"packageUris\":[\"http://schema.mathworks.com/mf0/Connector/R2020b\"],\"version\":\"1.0\"}"
  Chart5 : Stateflow chart  TreatAsAtomicUnit=on
      settings: PortSchema="{\"entries\":[{\"content\":{\"sides\":[{\"content\":{\"connectorIds\":[\"In1\",\"In2\",\"In3\",\"In4\",\"In5\"]},\"type\":\"ConnectorPlacement.EquallySpacedRectSide\",\"uuid\":\"0588d813-8053-43c2-aa9d-d3a846613814\"},{\"content\":{\"connectorIds\":[\"Out3\",\"Out1\",\"Out2\"],\"side\":\"RIGHT\"},\"type\":\"ConnectorPlacement.EquallySpacedRectSide\",\"uuid\":\"b273383a-6a54-4b9f-9eb1-40fc7adfc00e\"},{\"content\":{\"connectorIds\":[],\"side\":\"TOP\"},\"type\":\"ConnectorPlacement.EquallySpacedRectSide\",\"uuid\":\"d9b37716-6c8a-415a-a248-7c4c2a5acdca\"}]},\"type\":\"ConnectorPlacement.EquallySpacedConnector\",\"uuid\":\"4383e6fa-6fc5-4afb-a6cc-0c4f83dd9bd6\"}],\"packageUris\":[\"http://schema.mathworks.com/mf0/Connector/R2020b\"],\"version\":\"1.0\"}"
  Chart6 : Stateflow chart  TreatAsAtomicUnit=on
  Constant1 : Constant  Value=0.5
  Constant14 : Constant  Value=2
  Constant16 : Constant  Value=0
  Constant17 : Constant  Value=0
  Constant18 : Constant  Value=0
  Constant2 : Constant  Value=8
  Constant3 : Constant  Value=4.65
  Constant4 : Constant
  Constant9 : Constant  Value=3.35
  Demux1 : Demux  Outputs=3
  Demux3 : Demux  Outputs=3
  Demux5 : Demux  Outputs=3
  Display1 : Display
  Function Caller2 : FunctionCaller  FunctionPrototype=y = f(u)  InputArgumentSpecifications=<Enter example>  OutputArgumentSpecifications=<Enter example>
  Function Caller3 : FunctionCaller  FunctionPrototype=y = f(u)  InputArgumentSpecifications=<Enter example>  OutputArgumentSpecifications=<Enter example>
  If2 : If  IfExpression=u1 > 5.5
  MATLAB Function5 : MATLAB Function  TreatAsAtomicUnit=on
  MATLAB Function6 : MATLAB Function  TreatAsAtomicUnit=on
  MATLAB Function7 : MATLAB Function  TreatAsAtomicUnit=on
  MATLAB Function8 : MATLAB Function  TreatAsAtomicUnit=on
  MATLAB Function9 : MATLAB Function  TreatAsAtomicUnit=on
  Matrix Concatenate1 : Concatenate  Mode=Multidimensional array  ConcatenateDimension=2
  Mod2 : Math  Operator=mod  SaturateOnIntegerOverflow=on
  Mux2 : Mux  Inputs=2
  Mux3 : Mux  Inputs=2
  Pi2 : Constant  Value=pi  OutDataTypeStr=Inherit: Inherit via back propagation
  Product1 : Product
  Proximity_Finder_Ball3 : Subsystem
  Proximity_Finder_Ball4 : Subsystem
  Simulink Function1 : Subsystem  TreatAsAtomicUnit=on
  Subsystem3 : Subsystem
  Subsystem4 : Subsystem
  Sum1 : Sum  Inputs=+-
  Sum5 : Sum  Inputs=-+
  Sum6 : Sum  Inputs=-+
  Switch3 : Switch  Criteria=u2 > Threshold
  Switch4 : Switch  Criteria=u2 > Threshold
  Unit Delay1 : UnitDelay  SampleTime=-1  HasFrameUpgradeWarning=on
  Vector Concatenate1 : Concatenate  NumInputs=3
  Vector Concatenate2 : Concatenate
  kickForceSim1 : FromWorkspace  Commented=on  VariableName=out.KickForce
  kick_direction2 : Subsystem
  min_Distance_Finder1 : Subsystem
      settings: PortSchema="{\"entries\":[{\"content\":{\"sides\":[{\"content\":{\"connectorIds\":[\"In1\",\"In2\"]},\"type\":\"ConnectorPlacement.EquallySpacedRectSide\",\"uuid\":\"45cf91c7-7d38-4a19-bf35-d1d31095287a\"},{\"content\":{\"connectorIds\":[\"Out1\",\"Out2\",\"Out3\",\"Out4\"],\"side\":\"RIGHT\"},\"type\":\"ConnectorPlacement.EquallySpacedRectSide\",\"uuid\":\"645394ba-2e5d-4060-b61c-cc9330ee0038\"},{\"content\":{\"connectorIds\":[\"In3\",\"In4\",\"In5\"],\"side\":\"TOP\"},\"type\":\"ConnectorPlacement.EquallySpacedRectSide\",\"uuid\":\"4fc56b73-04ec-476f-b487-f0e593f708ad\"},{\"content\":{\"connectorIds\":[],\"side\":\"BOTTOM\"},\"type\":\"ConnectorPlacement.EquallySpacedRectSide\",\"uuid\":\"cd306436-fd63-4e79-88e6-7a63c0840ed7\"}]},\"type\":\"ConnectorPlacement.EquallySpacedConnector\",\"uuid\":\"5cf2ee04-00eb-490b-958c-5fb90b43d325\"}],\"packageUris\":[\"http://schema.mathworks.com/mf0/Connector/R2020b\"],\"version\":\"1.0\"}"
  XYZK : Outport
  VxVyW : Outport  Port=2
  wires:
  Sum6/1 -> Proximity_Finder_Ball4/1(In1)
  Robot 6 T1 Loc3/1 -> MATLAB Function7/2(r3), min_Distance_Finder1/4(R_3_loc)
  Demux1/2 -> MATLAB Function8/2(goal_keeperY)
  Chart5/2(velocity) -> Chart6/1(velocity)
  Constant2/1 -> MATLAB Function5/1(F)
  Robot 1 T1 Loc/1 -> min_Distance_Finder1/2(R_2_loc), MATLAB Function6/4(rob_loc), Demux3/1
  Angle Finder2/1(angle) -> Chart3/5(angle)
  Demux5/1 -> Vector Concatenate2/1, Subsystem4/2(In2), If2/1
  min_Distance_Finder1/4(nearest_robot) -> Chart5/5(nearest_rob)
  Sum1/1 -> Proximity_Finder_Ball3/1(In1), Angle Finder2/1(In1)
  Vector Concatenate1/1 -> VxVyW/1
  MATLAB Function6/2(z) -> Sum5/1
  Unit Delay1/1 -> [A]
  Matrix Concatenate1/1 -> Sum6/2, Sum5/2, Sum1/1
  Pi2/1 -> Product1/1
  Vector Concatenate2/1 -> Sum1/2
  Robot 5 T1 Loc4/1 -> Demux1/1, min_Distance_Finder1/3(R_1_loc)
  MATLAB Function6/1(y) -> MATLAB Function5/2(dis)
  MATLAB Function5/1(dF) -> kick_direction2/3(dF)
  Constant16/1 -> Vector Concatenate1/2
  Function Caller2/1 -> MATLAB Function8/1(distance_to_goal1)
  Chart6/2(w) -> Vector Concatenate1/3
  Product1/1 -> Mod2/2
  Constant4/1 -> Mux3/1, Mux2/1
  Robot 8 T1 Loc2/1 -> MATLAB Function7/3(r4), min_Distance_Finder1/5(R_4_loc)
  min_Distance_Finder1/1(nearest_team) -> Chart5/2(nearest_team), MATLAB Function6/3(team), Display1/1
  Ball Loc/1 -> Demux5/1
  min_Distance_Finder1/3(nearest_team_idx) -> MATLAB Function7/1(u)
  min_Distance_Finder1/2(nearest_opponent) -> Chart5/3(nearest_op)
  Sum5/1 -> kick_direction2/1(In1)
  Constant9/1 -> Mux2/2
  Chart5/1(kick) -> Switch4/3
  Subsystem4/1(Out1) -> Chart3/1(Bx)
  Proximity_Finder_Ball4/1(DBR) -> MATLAB Function6/2(goal), Chart5/4(distance_to_goal)
  Mod2/1 -> Chart3/6(angle_bot)
  Mux2/1 -> Function Caller2/1
  Constant1/1 -> MATLAB Function5/3(dT)
  Proximity_Finder_Ball3/1(DBR) -> Chart5/1(distance_to_ball)
  Function Caller3/1 -> MATLAB Function8/3(distance_to_goal2)
  Chart6/1(v) -> Switch3/3
  Demux3/3 -> Mod2/1
  If2/1 -> Subsystem4/1(Action Port)
  Chart3/1(actual_angle) -> Chart6/2(DT)
  Robot 7 sens/1 -> min_Distance_Finder1/1(R_2_sen)
  Demux3/1 -> Matrix Concatenate1/1, Chart3/3(Rx)
  MATLAB Function9/1(y) -> Unit Delay1/1
  MATLAB Function7/1(y) -> MATLAB Function6/5(rob_loc1)
  Constant3/1 -> Mux3/2
  Subsystem3/1(Out1) -> Sum6/1
  kick_direction2/1(XYZK) -> XYZK/1
  Demux5/2 -> Chart3/2(By), Vector Concatenate2/2
  Demux3/2 -> Matrix Concatenate1/2, Chart3/4(Ry)
  Constant14/1 -> Product1/2
  Mux3/1 -> Function Caller3/1
  If2/2 -> Subsystem4/3(Action Port1)
  MATLAB Function8/1(centroid) -> [centroid]
  Chart5/3(pass_beh) -> MATLAB Function9/1(u), MATLAB Function6/1(beh)
  Constant17/1 -> Switch3/1
  Switch3/1 -> Vector Concatenate1/1
  velocity_UA/1 -> Switch3/2
  Constant18/1 -> Switch4/1
  Switch4/1 -> kick_direction2/2(kick)
  kick_UA/1 -> Switch4/2

== system Control_try_final_2020b/Team_1_behaviour/T1R1(Goal_Keeper)/Ball_in_D/Angle Finder ==
  In1 : Inport
  Abs : Abs
  Atan : Trigonometry  Operator=atan
  Demux : Demux  Outputs=2
  Divide : Product  Inputs=/*
  angle : Outport
  wires:
  Divide/1 -> Atan/1
  Demux/2 -> Divide/2
  Demux/1 -> Divide/1
  Atan/1 -> Abs/1
  Abs/1 -> angle/1
  In1/1 -> Demux/1

== system Control_try_final_2020b/Team_1_behaviour/T1R1(Goal_Keeper)/Ball_in_D/Proximity_Finder_Ball ==
  In1 : Inport
  Demux : Demux  Outputs=2
  Sqrt : Sqrt  SaturateOnIntegerOverflow=on
  Square : Math  Operator=square  SaturateOnIntegerOverflow=on
  Square1 : Math  Operator=square  SaturateOnIntegerOverflow=on
  Sum : Sum
  DBR : Outport
  wires:
  In1/1 -> Demux/1
  Demux/1 -> Square/1
  Demux/2 -> Square1/1
  Square1/1 -> Sum/2
  Square/1 -> Sum/1
  Sum/1 -> Sqrt/1
  Sqrt/1 -> DBR/1

== system Control_try_final_2020b/Team_1_behaviour/T1R1(Goal_Keeper)/Ball_in_D/kick_direction ==
  In1 : Inport
  kick : Inport  Port=2
  Angle Finder1 : Subsystem
  Chart1 : Stateflow chart  TreatAsAtomicUnit=on
  Chart2 : Stateflow chart  TreatAsAtomicUnit=on
  Constant : Constant  Value=2.5
  Constant1 : Constant  Value=2.5
  Constant2 : Constant
  Cos : Trigonometry  Operator=cos
  Demux2 : Demux  Outputs=2
  Product : Product  Inputs=3
  Product1 : Product  Inputs=3
  Sin : Trigonometry
  Vector Concatenate : Concatenate  NumInputs=4
  Out1 : Outport
  wires:
  Demux2/2 -> Chart2/1(y)
  Demux2/1 -> Chart1/1(x)
  In1/1 -> Angle Finder1/1(In1), Demux2/1
  Chart1/1(Vx) -> Product/2
  Cos/1 -> Product/3
  Angle Finder1/1(angle) -> Cos/1, Sin/1
  Constant/1 -> Product/1
  Constant1/1 -> Product1/3
  Chart2/1(Vy) -> Product1/2
  Sin/1 -> Product1/1
  Product/1 -> Vector Concatenate/1
  Product1/1 -> Vector Concatenate/2
  Constant2/1 -> Vector Concatenate/3
  kick/1 -> Vector Concatenate/4
  Vector Concatenate/1 -> Out1/1

== system Control_try_final_2020b/Team_1_behaviour/T1R1(Goal_Keeper)/ball_out_of_D/Distance ==
  In1 : Inport
  In2 : Inport  Port=2
  In3 : Inport  Port=3
  In4 : Inport  Port=4
  Square : Math  Operator=square  SaturateOnIntegerOverflow=on
  Square Root : Sqrt  SaturateOnIntegerOverflow=on
  Square1 : Math  Operator=square  SaturateOnIntegerOverflow=on
  Sum : Sum  Inputs=|+-
  Sum1 : Sum  Inputs=|+-
  Sum2 : Sum  Inputs=|++
  GB_dist : Outport
  wires:
  Square1/1 -> Sum2/2
  Sum2/1 -> Square Root/1
  Square/1 -> Sum2/1
  Sum1/1 -> Square1/1
  Sum/1 -> Square/1
  In1/1 -> Sum/1
  In3/1 -> Sum/2
  In2/1 -> Sum1/1
  In4/1 -> Sum1/2
  Square Root/1 -> GB_dist/1

== system Control_try_final_2020b/Team_1_behaviour/T1R1(Goal_Keeper)/ball_out_of_D/Subsystem ==
  kick_direction : Inport
  R_1_loc : Inport  Port=2
  kick : Inport  Port=3
  Atan : Trigonometry  Operator=atan
  Constant : Constant  Value=2.5
  Constant1 : Constant  Value=2.5
  Constant2 : Constant  Value=0
  Cos : Trigonometry  Operator=cos
  Demux : Demux  Outputs=3
  Divide : Product  Inputs=/*
  Product : Product
  Product1 : Product
  Sin : Trigonometry
  Sum : Sum  Inputs=|+-
  Vector Concatenate : Concatenate  NumInputs=4
  Out1 : Outport  PortDimensions=4
  wires:
  Sum/1 -> Demux/1
  Constant1/1 -> Product1/2
  Sin/1 -> Product1/1
  Divide/1 -> Atan/1
  Demux/1 -> Divide/1
  Atan/1 -> Cos/1, Sin/1
  Product/1 -> Vector Concatenate/1
  Demux/2 -> Divide/2
  Constant2/1 -> Vector Concatenate/3
  Product1/1 -> Vector Concatenate/2
  kick/1 -> Vector Concatenate/4
  kick_direction/1 -> Sum/1
  R_1_loc/1 -> Sum/2
  Vector Concatenate/1 -> Out1/1
  Constant/1 -> Product/1
  Cos/1 -> Product/2

== system Control_try_final_2020b/Team_1_behaviour/T1R1(Goal_Keeper)/min_Distance_Finder/Distance ==
  R_1_loc : Inport
  R_2_loc : Inport  Port=2
  Demux : Demux  Outputs=3
  Demux1 : Demux  Outputs=3
  Square : Math  Operator=square  SaturateOnIntegerOverflow=on
  Square Root : Sqrt  SaturateOnIntegerOverflow=on
  Square1 : Math  Operator=square  SaturateOnIntegerOverflow=on
  Sum : Sum  Inputs=|+-
  Sum1 : Sum  Inputs=|+-
  Sum2 : Sum  Inputs=|++
  R1_R2_dis : Outport
  wires:
  Square1/1 -> Sum2/2
  Demux/2 -> Sum1/1
  Sum2/1 -> Square Root/1
  Square/1 -> Sum2/1
  Demux/1 -> Sum/1
  Sum1/1 -> Square1/1
  Demux1/2 -> Sum1/2
  Sum/1 -> Square/1
  Demux1/1 -> Sum/2
  R_1_loc/1 -> Demux/1
  R_2_loc/1 -> Demux1/1
  Square Root/1 -> R1_R2_dis/1

== system Control_try_final_2020b/Team_1_behaviour/T1R1(Goal_Keeper)/min_Distance_Finder/Distance1 ==
  R_1_loc : Inport
  R_3_loc : Inport  Port=2
  Demux : Demux  Outputs=3
  Demux1 : Demux  Outputs=3
  Square : Math  Operator=square  SaturateOnIntegerOverflow=on
  Square Root : Sqrt  SaturateOnIntegerOverflow=on
  Square1 : Math  Operator=square  SaturateOnIntegerOverflow=on
  Sum : Sum  Inputs=|+-
  Sum1 : Sum  Inputs=|+-
  Sum2 : Sum  Inputs=|++
  R1_R3_dis : Outport
  wires:
  Square1/1 -> Sum2/2
  Demux/2 -> Sum1/1
  Sum2/1 -> Square Root/1
  Square/1 -> Sum2/1
  Demux/1 -> Sum/1
  Sum1/1 -> Square1/1
  Demux1/2 -> Sum1/2
  Sum/1 -> Square/1
  Demux1/1 -> Sum/2
  R_1_loc/1 -> Demux/1
  R_3_loc/1 -> Demux1/1
  Square Root/1 -> R1_R3_dis/1

== system Control_try_final_2020b/Team_1_behaviour/T1R1(Goal_Keeper)/min_Distance_Finder/Distance2 ==
  R_1_loc : Inport
  R_4_loc : Inport  Port=2
  Demux : Demux  Outputs=3
  Demux1 : Demux  Outputs=3
  Square : Math  Operator=square  SaturateOnIntegerOverflow=on
  Square Root : Sqrt  SaturateOnIntegerOverflow=on
  Square1 : Math  Operator=square  SaturateOnIntegerOverflow=on
  Sum : Sum  Inputs=|+-
  Sum1 : Sum  Inputs=|+-
  Sum2 : Sum  Inputs=|++
  R1_R4_dis : Outport
  wires:
  Square1/1 -> Sum2/2
  Demux/2 -> Sum1/1
  Sum2/1 -> Square Root/1
  Square/1 -> Sum2/1
  Demux/1 -> Sum/1
  Sum1/1 -> Square1/1
  Demux1/2 -> Sum1/2
  Sum/1 -> Square/1
  Demux1/1 -> Sum/2
  R_1_loc/1 -> Demux/1
  R_4_loc/1 -> Demux1/1
  Square Root/1 -> R1_R4_dis/1

== system Control_try_final_2020b/Team_1_behaviour/T1R1(Goal_Keeper)/min_Distance_Finder/R2_O_dist_val ==
  R_1_loc : Inport
  R_2_loc : Inport  Port=2
  sen_1_val : Inport  Port=3
  Chart : Stateflow chart  TreatAsAtomicUnit=on
  y : Outport
  wires:
  sen_1_val/1 -> Chart/2(sen_1_val)
  R_1_loc/1 -> Chart/1(R_1_loc)
  R_2_loc/1 -> Chart/3(R_2_loc)
  Chart/1(dist) -> y/1

== system Control_try_final_2020b/Team_1_behaviour/T1R1(Goal_Keeper)/min_Distance_Finder/R3_O_dist_val ==
  R_1_loc : Inport
  R_2_loc : Inport  Port=2
  sen_1_val : Inport  Port=3
  Chart : Stateflow chart  TreatAsAtomicUnit=on
  y : Outport
  wires:
  Chart/1(dist) -> y/1
  R_2_loc/1 -> Chart/3(R_2_loc)
  R_1_loc/1 -> Chart/1(R_1_loc)
  sen_1_val/1 -> Chart/2(sen_1_val)

== system Control_try_final_2020b/Team_1_behaviour/T1R1(Goal_Keeper)/min_Distance_Finder/R4_O_dist_val ==
  R_1_loc : Inport
  R_2_loc : Inport  Port=2
  sen_1_val : Inport  Port=3
  Chart : Stateflow chart  TreatAsAtomicUnit=on
  y : Outport
  wires:
  sen_1_val/1 -> Chart/2(sen_1_val)
  R_1_loc/1 -> Chart/1(R_1_loc)
  R_2_loc/1 -> Chart/3(R_2_loc)
  Chart/1(dist) -> y/1

== system Control_try_final_2020b/Team_1_behaviour/T1R2 (attacker 1)/Team 1 Behaviour1/Angle Finder1 ==
  In1 : Inport
  Abs : Abs
  Atan : Trigonometry  Operator=atan
  Demux : Demux  Outputs=2
  Divide : Product  Inputs=/*
  angle : Outport
  wires:
  Divide/1 -> Atan/1
  Demux/2 -> Divide/2
  Demux/1 -> Divide/1
  Atan/1 -> Abs/1
  Abs/1 -> angle/1
  In1/1 -> Demux/1

== system Control_try_final_2020b/Team_1_behaviour/T1R2 (attacker 1)/Team 1 Behaviour1/Proximity_Finder_Ball1 ==
  In1 : Inport
  Demux : Demux  Outputs=2
  Sqrt : Sqrt  SaturateOnIntegerOverflow=on
  Square : Math  Operator=square  SaturateOnIntegerOverflow=on
  Square1 : Math  Operator=square  SaturateOnIntegerOverflow=on
  Sum : Sum
  DBR : Outport
  wires:
  In1/1 -> Demux/1
  Demux/1 -> Square/1
  Demux/2 -> Square1/1
  Square1/1 -> Sum/2
  Square/1 -> Sum/1
  Sum/1 -> Sqrt/1
  Sqrt/1 -> DBR/1

== system Control_try_final_2020b/Team_1_behaviour/T1R2 (attacker 1)/Team 1 Behaviour1/Proximity_Finder_Ball2 ==
  In1 : Inport
  Demux : Demux  Outputs=2
  Sqrt : Sqrt  SaturateOnIntegerOverflow=on
  Square : Math  Operator=square  SaturateOnIntegerOverflow=on
  Square1 : Math  Operator=square  SaturateOnIntegerOverflow=on
  Sum : Sum
  DBR : Outport
  wires:
  Sqrt/1 -> DBR/1
  Sum/1 -> Sqrt/1
  Square/1 -> Sum/1
  Square1/1 -> Sum/2
  Demux/2 -> Square1/1
  Demux/1 -> Square/1
  In1/1 -> Demux/1

== system Control_try_final_2020b/Team_1_behaviour/T1R2 (attacker 1)/Team 1 Behaviour1/Simulink Function ==
  f : TriggerPort  TriggerType=function-call  IsSimulinkFunction=on  FunctionName=f  FunctionVisibility=scoped  VariantControl=(inherit)
  Demux : Demux  Outputs=2
  Sqrt : Sqrt  SaturateOnIntegerOverflow=on
  Square : Math  Operator=square  SaturateOnIntegerOverflow=on
  Square1 : Math  Operator=square  SaturateOnIntegerOverflow=on
  Sum : Sum
  u : ArgIn  DisableCoverage=on  PortDimensions=[1 2]  ArgumentName=u
  y : ArgOut  DisableCoverage=on  ArgumentName=y
  wires:
  u/1 -> Demux/1
  Square/1 -> Sum/1
  Sum/1 -> Sqrt/1
  Sqrt/1 -> y/1
  Square1/1 -> Sum/2
  Demux/1 -> Square/1
  Demux/2 -> Square1/1
